simulink model "UOIT_EV_2016b"  (R2016b)
settings: Solver=VariableStepAuto  StartTime=0.0  StopTime=1  RelTol=1e-3
model workspace (MAT data in the model file):
  AccessoryLoad = 600
  C_ref = 600
  DrCycles : struct (value not decoded)
  K = 1.04716227018
  Kc_ref = 0.12
  Ki_ref = 0.01
  Kw_ref = 1.2e-05
  MDL : struct (value not decoded)
  T_max = 500
  T_ref = 300
  TimeHWFET = 765
  TimeUDDS = 1372
  TimeUS06 = 596
  aeroDragCoeff = 0.38
  airDensity = 1.23
  energyCapacity = 12.6
  frontArea = 2.1
  gravity = 9.81
  inclinationAngle = 0
  inertialMassVeh = 2392
  initialSOC = 0.95
  internalResistance = 0.1
  massVeh = 2300
  openCircuitVoltage = 340
  rollingResistCoeff = 0.01
  w_max = 524
  w_ref = 834
  wheelRadius = 0.34
libraries: autolibmotorctrlr x4, simulink x3
(part 3 of 3)

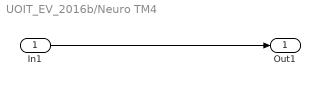
== system UOIT_EV_2016b/Neuro TM4 ==
  In1 : Inport
  Out1 : Outport
  wires:
  In1/1 -> Out1/1

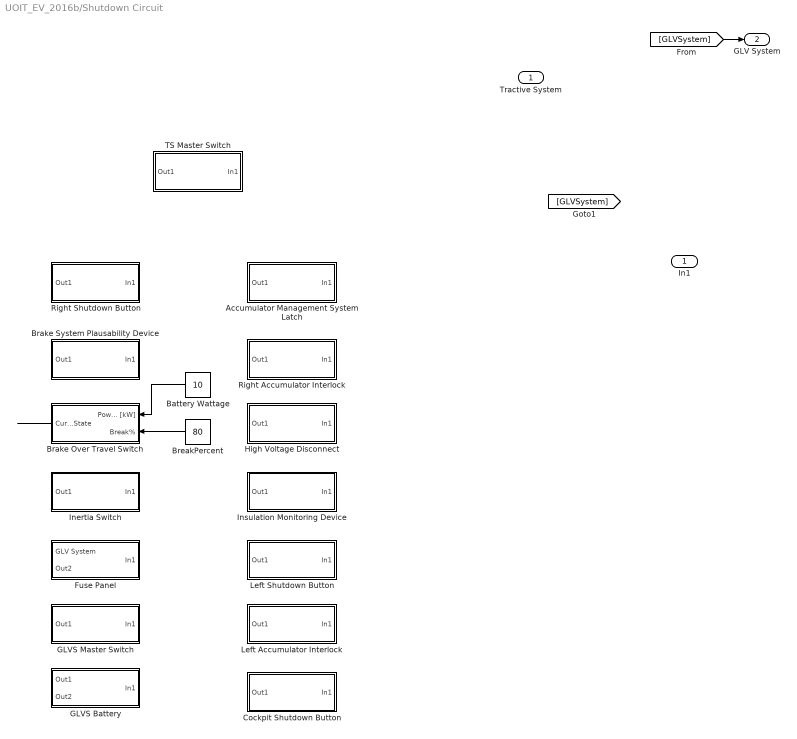
== system UOIT_EV_2016b/Shutdown Circuit ==
  In1 : Inport
  Accumulator Management System Latch : Subsystem
  Battery Wattage : Constant  Value=10
  Brake Over Travel Switch : Subsystem
  Brake System Plausability Device : Subsystem
  BreakPercent : Constant  Value=80
  Cockpit Shutdown Button : Subsystem
  Fuse Panel : Subsystem
  GLVS Battery : Subsystem
  GLVS Master Switch : Subsystem
  High Voltage Disconnect : Subsystem
  Inertia Switch : Subsystem
  Insulation Monitoring Device : Subsystem
  Left Accumulator Interlock : Subsystem
  Left Shutdown Button : Subsystem
  Right Accumulator Interlock : Subsystem
  Right Shutdown Button : Subsystem
  TS Master Switch : Subsystem
  Tractive System : Outport
  GLV System : Outport  Port=2
  wires:
  [GLVSystem] -> GLV System/1
  Battery Wattage/1 -> Brake Over Travel Switch/1(Power [kW])
  BreakPercent/1 -> Brake Over Travel Switch/2(Break%)
  Brake Over Travel Switch/1(CurrentState) -> ?

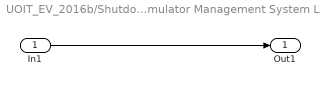
== system UOIT_EV_2016b/Shutdown Circuit/Accumulator Management System Latch ==
  In1 : Inport
  Out1 : Outport
  wires:
  In1/1 -> Out1/1

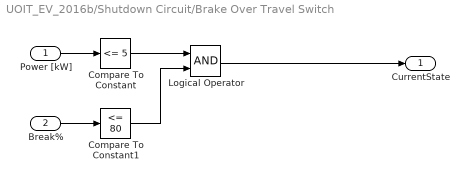
== system UOIT_EV_2016b/Shutdown Circuit/Brake Over Travel Switch ==
  Power [kW] : Inport
  Break% : Inport  Port=2
  Compare To Constant : simulink/Logic and Bit Operations/Compare To Constant  relop=<=  const=5  OutDataTypeStr=boolean
  Compare To Constant1 : simulink/Logic and Bit Operations/Compare To Constant  relop=<=  const=80  OutDataTypeStr=boolean
  Logical Operator : Logic  AllPortsSameDT=off  OutDataTypeStr=boolean
  CurrentState : Outport
  wires:
  Break%/1 -> Compare To Constant1/1
  Power [kW]/1 -> Compare To Constant/1
  Compare To Constant1/1 -> Logical Operator/2
  Compare To Constant/1 -> Logical Operator/1
  Logical Operator/1 -> CurrentState/1

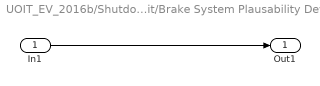
== system UOIT_EV_2016b/Shutdown Circuit/Brake System Plausability Device ==
  In1 : Inport
  Out1 : Outport
  wires:
  In1/1 -> Out1/1

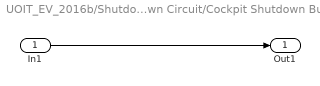
== system UOIT_EV_2016b/Shutdown Circuit/Cockpit Shutdown Button ==
  In1 : Inport
  Out1 : Outport
  wires:
  In1/1 -> Out1/1

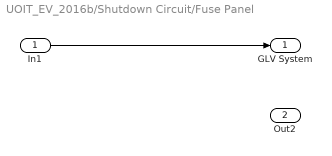
== system UOIT_EV_2016b/Shutdown Circuit/Fuse Panel ==
  In1 : Inport
  GLV System : Outport
  Out2 : Outport  Port=2
  wires:
  In1/1 -> GLV System/1

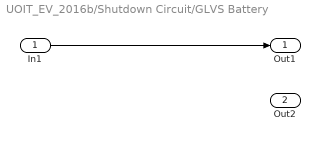
== system UOIT_EV_2016b/Shutdown Circuit/GLVS Battery ==
  In1 : Inport
  Out1 : Outport
  Out2 : Outport  Port=2
  wires:
  In1/1 -> Out1/1

== system UOIT_EV_2016b/Shutdown Circuit/GLVS Master Switch ==
  In1 : Inport
  Out1 : Outport
  wires:
  In1/1 -> Out1/1

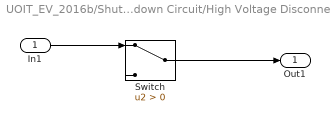
== system UOIT_EV_2016b/Shutdown Circuit/High Voltage Disconnect ==
  In1 : Inport
  Switch : Switch  Criteria=u2 > Threshold
  Out1 : Outport
  wires:
  In1/1 -> Switch/1
  Switch/1 -> Out1/1

== system UOIT_EV_2016b/Shutdown Circuit/Inertia Switch ==
  In1 : Inport
  Out1 : Outport
  wires:
  In1/1 -> Out1/1

== system UOIT_EV_2016b/Shutdown Circuit/Insulation Monitoring Device ==
  In1 : Inport
  Out1 : Outport
  wires:
  In1/1 -> Out1/1

== system UOIT_EV_2016b/Shutdown Circuit/Left Accumulator Interlock ==
  In1 : Inport
  Out1 : Outport
  wires:
  In1/1 -> Out1/1

== system UOIT_EV_2016b/Shutdown Circuit/Left Shutdown Button ==
  In1 : Inport
  Out1 : Outport
  wires:
  In1/1 -> Out1/1

== system UOIT_EV_2016b/Shutdown Circuit/Right Accumulator Interlock ==
  In1 : Inport
  Out1 : Outport
  wires:
  In1/1 -> Out1/1

== system UOIT_EV_2016b/Shutdown Circuit/Right Shutdown Button ==
  In1 : Inport
  Out1 : Outport
  wires:
  In1/1 -> Out1/1

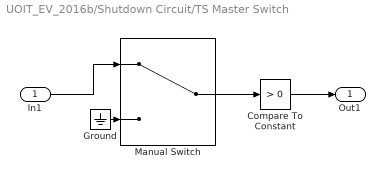
== system UOIT_EV_2016b/Shutdown Circuit/TS Master Switch ==
  In1 : Inport
  Compare To Constant : simulink/Logic and Bit Operations/Compare To Constant  relop=>  const=0  OutDataTypeStr=boolean
  Ground : Ground
  Manual Switch : ManualSwitch
  Out1 : Outport
  wires:
  In1/1 -> Manual Switch/1
  Ground/1 -> Manual Switch/2
  Compare To Constant/1 -> Out1/1
  Manual Switch/1 -> Compare To Constant/1
